simulink model "project"  (R2022b)
settings: Solver=FixedStepAuto  StartTime=0.0  StopTime=inf  RelTol=1e-3  EnableMultiTasking=on
libraries: arduinolib x10
settings Model: ExtModeTrigDuration=2  Creator=ESE  LastModifiedBy=ESE
settings OptimizationCC: EnhancedBackFolding=on  PassReuseOutputArgsAs=Individual arguments  ZeroExternalMemoryAtStartup=off  ZeroInternalMemoryAtStartup=off  MaxStackSize=64  OptimizeBlockOrder=speed  DifferentSizesBufferReuse=on  OptimizationCustomize=off  EfficientTunableParamExpr=on
settings DebuggingCC: ParameterTunabilityLossMsg=error
settings HardwareCC: ProdBitPerInt=16  ProdBitPerPointer=16  ProdBitPerSizeT=16  ProdBitPerPtrDiffT=16  ProdLargestAtomicFloat=None  ProdWordSize=8  ProdHWDeviceType=Atmel->AVR
settings SFSimCC: MATLABDynamicMemAlloc=off
settings RTWCC: Description=Embedded Coder  SystemTargetFile=ert.tlc  HardwareBoard=Arduino Mega 2560  TLCOptions=-aInlineSetEventsForThisBaseRateFcn=TLC_FALSE -aSuppressMultiTaskScheduler=TLC_FALSE -aRateBasedStepFcn=1  TemplateMakefile=ert_default_tmf  Toolchain=Arduino AVR  BuildConfiguration=Faster Runs
settings CodeAppCC: ForceParamTrailComments=on  IgnoreCustomStorageClasses=off  OperatorAnnotations=on  SimulinkDataObjDesc=on  SFDataObjDesc=on  InsertBlockDesc=on
settings ERTTargetCC: SupportContinuousTime=on  SupportVariableSizeSignals=on  ExtModeTransport=3  ExtModeStaticAlloc=on  ExtModeAutomaticAllocSize=off  ExtModeStaticAllocSize=2048  ExtModeMexFile=ext_xcp  ExtModeIntrfLevel=Level2 - Open

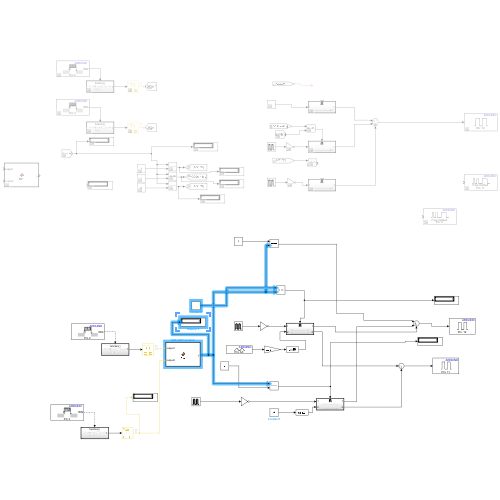
[thumbnail: Simulink's stored preview of the top-level diagram]
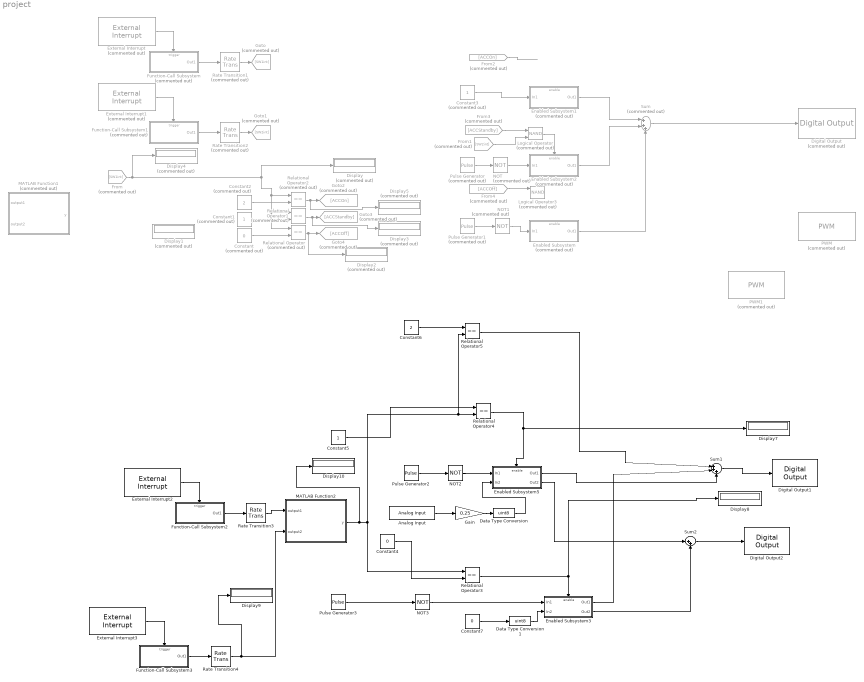
== system project ==
  Analog Input : arduinolib/Analog Input  pinNumber=0  ReadResultsOnly=off  ConversionTriggerSource=Software  ExternalTriggerType=uint32( 0 )  OutputDataType=uint16  EnableConversionCompleteNotify=off  EnableOuputStatus=off  SampleTime=-1  blockPlatform=arduino
  Constant : Constant  Commented=on  Value=0
  Constant1 : Constant  Commented=on
  Constant2 : Constant  Commented=on  Value=2
  Constant3 : Constant  Commented=on
  Constant4 : Constant  Value=0
  Constant5 : Constant
  Constant6 : Constant  Value=2
  Constant7 : Constant  Value=0
  Data Type Conversion : DataTypeConversion  OutDataTypeStr=uint8  SaturateOnIntegerOverflow=off  RndMeth=Floor
  Data Type Conversion1 : DataTypeConversion  OutDataTypeStr=uint8  SaturateOnIntegerOverflow=off  RndMeth=Floor
  Digital Output : arduinolib/Digital Output  Commented=on  pinNumber=12  Direction=output  blockPlatform=arduino
  Digital Output1 : arduinolib/Digital Output  pinNumber=12  Direction=output  blockPlatform=arduino
  Digital Output2 : arduinolib/Digital Output  pinNumber=11  Direction=output  blockPlatform=arduino
  Display{,1..5} (6 alike) : Display  Commented=on
  Display{7..10} (4 alike) : Display
  Enabled Subsystem : Subsystem  Commented=on  TreatAsAtomicUnit=on
  Enabled Subsystem1 : Subsystem  Commented=on  TreatAsAtomicUnit=on
  Enabled Subsystem2 : Subsystem  Commented=on  TreatAsAtomicUnit=on
  Enabled Subsystem3 : Subsystem  TreatAsAtomicUnit=on
  Enabled Subsystem5 : Subsystem  TreatAsAtomicUnit=on
  External Interrupt : arduinolib/External Interrupt  Commented=on  Pin=2  PullUp=off  Mode=FALLING  InterruptSimulationInput=off
  External Interrupt1 : arduinolib/External Interrupt  Commented=on  Pin=3  PullUp=off  Mode=FALLING  InterruptSimulationInput=off
  External Interrupt2 : arduinolib/External Interrupt  Pin=2  PullUp=off  Mode=FALLING  InterruptSimulationInput=off
  External Interrupt3 : arduinolib/External Interrupt  Pin=3  PullUp=off  Mode=FALLING  InterruptSimulationInput=off
  From : From  Commented=on  GotoTag=SW1int
  From1 : From  Commented=on  GotoTag=SW2int
  From2 : From  Commented=on  GotoTag=ACCOn
  From3 : From  Commented=on  GotoTag=ACCStandby
  From4 : From  Commented=on  GotoTag=ACCOff
  Function-Call Subsystem : Subsystem  Commented=on  TreatAsAtomicUnit=on
  Function-Call Subsystem1 : Subsystem  Commented=on  TreatAsAtomicUnit=on
  Function-Call Subsystem2 : Subsystem  TreatAsAtomicUnit=on
  Function-Call Subsystem3 : Subsystem  TreatAsAtomicUnit=on
  Gain : Gain  Gain=0.25
  Goto : Goto  Commented=on  GotoTag=SW1int
  Goto1 : Goto  Commented=on  GotoTag=SW2int
  Goto2 : Goto  Commented=on  GotoTag=ACCOn
  Goto3 : Goto  Commented=on  GotoTag=ACCStandby
  Goto4 : Goto  Commented=on  GotoTag=ACCOff
  Logical Operator : Logic  Commented=on  Operator=NAND  AllPortsSameDT=off  OutDataTypeStr=boolean
  Logical Operator3 : Logic  Commented=on  Operator=NAND  AllPortsSameDT=off  OutDataTypeStr=boolean
  MATLAB Function1 : MATLAB Function  Commented=on  TreatAsAtomicUnit=on
  MATLAB Function2 : MATLAB Function  TreatAsAtomicUnit=on
  NOT : Logic  Commented=on  Operator=NOT  IconShape=distinctive  AllPortsSameDT=off  OutDataTypeStr=boolean
  NOT1 : Logic  Commented=on  Operator=NOT  IconShape=distinctive  AllPortsSameDT=off  OutDataTypeStr=boolean
  NOT2 : Logic  Operator=NOT  IconShape=distinctive  AllPortsSameDT=off  OutDataTypeStr=boolean
  NOT3 : Logic  Operator=NOT  IconShape=distinctive  AllPortsSameDT=off  OutDataTypeStr=boolean
  PWM : arduinolib/PWM  Commented=on  pinNumber=11  frequencyType=Default  desiredFrequency=490.2  achievableFrequency=490.2
  PWM1 : arduinolib/PWM  Commented=on  pinNumber=8  frequencyType=Default  desiredFrequency=490.2  achievableFrequency=490.2
  Pulse Generator : DiscretePulseGenerator  Commented=on  PulseType=Time based  Period=0.4  PulseWidth=50
  Pulse Generator1 : DiscretePulseGenerator  Commented=on  PulseType=Time based  Period=0.4  PulseWidth=50
  Pulse Generator2 : DiscretePulseGenerator  PulseType=Time based  Period=0.4  PulseWidth=50
  Pulse Generator3 : DiscretePulseGenerator  PulseType=Time based  Period=0.4  PulseWidth=50
  Rate Transition1 : RateTransition  Commented=on  Deterministic=off
  Rate Transition2 : RateTransition  Commented=on  Deterministic=off
  Rate Transition3 : RateTransition  Deterministic=off
  Rate Transition4 : RateTransition  Deterministic=off
  Relational Operator : RelationalOperator  Commented=on  Operator===  OutDataTypeStr=boolean  RndMeth=Simplest  InputSameDT=off
  Relational Operator1 : RelationalOperator  Commented=on  Operator===  OutDataTypeStr=boolean  RndMeth=Simplest  InputSameDT=off
  Relational Operator2 : RelationalOperator  Commented=on  Operator===  OutDataTypeStr=boolean  RndMeth=Simplest  InputSameDT=off
  Relational Operator3 : RelationalOperator  Operator===  OutDataTypeStr=boolean  RndMeth=Simplest  InputSameDT=off
  Relational Operator4 : RelationalOperator  Operator===  OutDataTypeStr=boolean  RndMeth=Simplest  InputSameDT=off
  Relational Operator5 : RelationalOperator  Operator===  OutDataTypeStr=boolean  RndMeth=Simplest  InputSameDT=off
  Sum : Sum  Commented=on  Inputs=|+++
  Sum1 : Sum  Inputs=|+++
  Sum2 : Sum  Inputs=|++
  wires:
  Rate Transition1/1 -> Goto/1
  Enabled Subsystem/1(Out1) -> Sum/3
  Function-Call Subsystem/1(Out1) -> Rate Transition1/1
  External Interrupt/1 -> Function-Call Subsystem/Trigger
  Constant3/1 -> Enabled Subsystem1/1(In1)
  Sum/1 -> Digital Output/1
  Pulse Generator1/1 -> NOT1/1
  Constant/1 -> Relational Operator/2
  Constant2/1 -> Relational Operator2/2
  Function-Call Subsystem1/1(Out1) -> Rate Transition2/1
  External Interrupt1/1 -> Function-Call Subsystem1/Trigger
  Relational Operator1/1 -> Display3/1, Goto3/1
  Relational Operator2/1 -> Display5/1, Goto2/1
  NOT/1 -> Enabled Subsystem2/1(In1)
  From/1 -> Relational Operator2/1, Relational Operator/1, Relational Operator1/1, Display/1, Display4/1
  NOT1/1 -> Enabled Subsystem/1(In1)
  Pulse Generator/1 -> NOT/1
  Rate Transition2/1 -> Goto1/1
  Relational Operator/1 -> Display2/1, Goto4/1
  Constant1/1 -> Relational Operator1/2
  From3/1 -> Logical Operator/1
  From1/1 -> Logical Operator/2
  Logical Operator/1 -> Enabled Subsystem2/Enable
  From2/1 -> ?
  Enabled Subsystem1/1(Out1) -> Sum/1
  Enabled Subsystem2/1(Out1) -> Sum/2
  From4/1 -> Logical Operator3/1
  Relational Operator4/1 -> Enabled Subsystem5/Enable, Display7/1
  Enabled Subsystem5/1(Out1) -> Sum1/3
  Constant4/1 -> Relational Operator3/2
  Constant5/1 -> Relational Operator4/1
  Pulse Generator2/1 -> NOT2/1
  Sum1/1 -> Digital Output1/1
  NOT2/1 -> Enabled Subsystem5/1(In1)
  Pulse Generator3/1 -> NOT3/1
  Enabled Subsystem3/1(Out1) -> Sum1/2
  Function-Call Subsystem2/1(Out1) -> Rate Transition3/1
  External Interrupt2/1 -> Function-Call Subsystem2/Trigger
  Relational Operator3/1 -> Display8/1, Enabled Subsystem3/Enable
  Constant6/1 -> Relational Operator5/1
  NOT3/1 -> Enabled Subsystem3/1(In1)
  Relational Operator5/1 -> Sum1/1
  Function-Call Subsystem3/1(Out1) -> Rate Transition4/1
  External Interrupt3/1 -> Function-Call Subsystem3/Trigger
  Rate Transition4/1 -> Display9/1, MATLAB Function2/2(output2)
  Rate Transition3/1 -> MATLAB Function2/1(output1)
  MATLAB Function2/1(y) -> Display10/1, Relational Operator5/2, Relational Operator4/2, Relational Operator3/1
  Gain/1 -> Data Type Conversion/1
  Analog Input/1 -> Gain/1
  Data Type Conversion/1 -> Enabled Subsystem5/2(In2)
  Enabled Subsystem5/2(Out2) -> Sum2/1
  Sum2/1 -> Digital Output2/1
  Enabled Subsystem3/2(Out2) -> Sum2/2
  Constant7/1 -> Data Type Conversion1/1
  Data Type Conversion1/1 -> Enabled Subsystem3/2(In2)

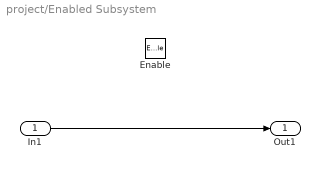
== system project/Enabled Subsystem ==
  In1 : Inport
  Enable : EnablePort  StatesWhenEnabling=reset
  Out1 : Outport
  wires:
  In1/1 -> Out1/1

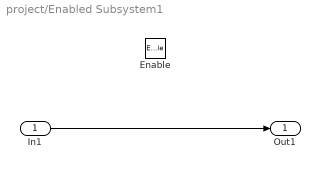
== system project/Enabled Subsystem1 ==
  In1 : Inport
  Enable : EnablePort
  Out1 : Outport
  wires:
  In1/1 -> Out1/1

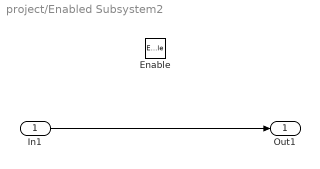
== system project/Enabled Subsystem2 ==
  In1 : Inport
  Enable : EnablePort
  Out1 : Outport
  wires:
  In1/1 -> Out1/1

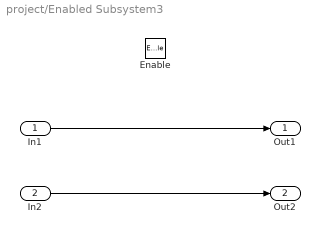
== system project/Enabled Subsystem3 ==
  In1 : Inport
  In2 : Inport  Port=2
  Enable : EnablePort  StatesWhenEnabling=reset
  Out1 : Outport
  Out2 : Outport  Port=2
  wires:
  In1/1 -> Out1/1
  In2/1 -> Out2/1

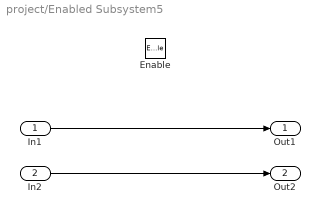
== system project/Enabled Subsystem5 ==
  In1 : Inport
  In2 : Inport  Port=2
  Enable : EnablePort
  Out1 : Outport
  Out2 : Outport  Port=2
  wires:
  In1/1 -> Out1/1
  In2/1 -> Out2/1

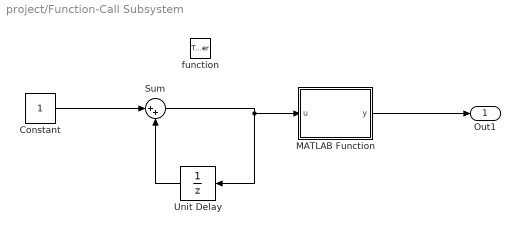
== system project/Function-Call Subsystem ==
  function : TriggerPort  TriggerType=function-call  VariantControl=(inherit)
  Constant : Constant
  MATLAB Function : MATLAB Function  TreatAsAtomicUnit=on
  Sum : Sum  Inputs=|++
  Unit Delay : UnitDelay  SampleTime=-1  HasFrameUpgradeWarning=on
  Out1 : Outport
  wires:
  Constant/1 -> Sum/1
  Unit Delay/1 -> Sum/2
  Sum/1 -> Unit Delay/1, MATLAB Function/1(u)
  MATLAB Function/1(y) -> Out1/1

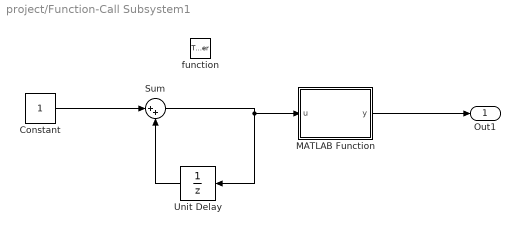
== system project/Function-Call Subsystem1 ==
  function : TriggerPort  TriggerType=function-call  VariantControl=(inherit)
  Constant : Constant
  MATLAB Function : MATLAB Function  TreatAsAtomicUnit=on
  Sum : Sum  Inputs=|++
  Unit Delay : UnitDelay  SampleTime=-1  HasFrameUpgradeWarning=on
  Out1 : Outport
  wires:
  Constant/1 -> Sum/1
  Unit Delay/1 -> Sum/2
  Sum/1 -> Unit Delay/1, MATLAB Function/1(u)
  MATLAB Function/1(y) -> Out1/1

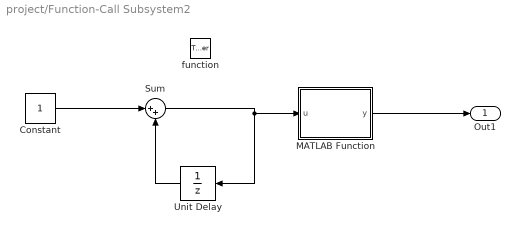
== system project/Function-Call Subsystem2 ==
  function : TriggerPort  TriggerType=function-call  VariantControl=(inherit)
  Constant : Constant
  MATLAB Function : MATLAB Function  TreatAsAtomicUnit=on
  Sum : Sum  Inputs=|++
  Unit Delay : UnitDelay  SampleTime=-1  HasFrameUpgradeWarning=on
  Out1 : Outport
  wires:
  Constant/1 -> Sum/1
  Unit Delay/1 -> Sum/2
  Sum/1 -> Unit Delay/1, MATLAB Function/1(u)
  MATLAB Function/1(y) -> Out1/1

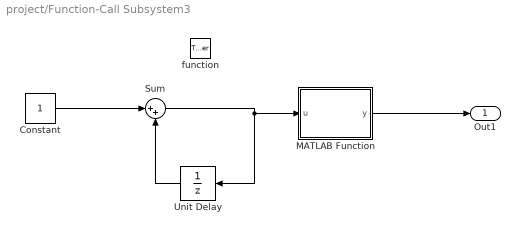
== system project/Function-Call Subsystem3 ==
  function : TriggerPort  TriggerType=function-call  VariantControl=(inherit)
  Constant : Constant
  MATLAB Function : MATLAB Function  TreatAsAtomicUnit=on
  Sum : Sum  Inputs=|++
  Unit Delay : UnitDelay  SampleTime=-1  HasFrameUpgradeWarning=on
  Out1 : Outport
  wires:
  Constant/1 -> Sum/1
  Unit Delay/1 -> Sum/2
  Sum/1 -> Unit Delay/1, MATLAB Function/1(u)
  MATLAB Function/1(y) -> Out1/1

== matlab function project/Function-Call Subsystem/MATLAB Function ==
  data: u input; y output
function y = fcn(u)
 rem = mod(u,3);

 if rem == 0
     y=0; %off
 elseif rem==1
     y=1; %ACC standard
 else 
     y=2; %ACC on
 end

 if u > 100
     u = 1;
 end

== matlab function project/Function-Call Subsystem2/MATLAB Function ==
  data: u input; y output
function y = fcn(u)
 rem = mod(u,3);

 if rem == 0
     y=0; %off
 elseif rem==1
     y=1; %ACC standard
 else 
     y=2; %ACC on
 end

 if u > 100
     u = 1;
 end

== matlab function project/MATLAB Function1 ==
  data: output1 input; y output; output2 input
function y = fcn(output1,output2)
if output2==0
    y=output1;
else
    y=0;
end

== matlab function project/Function-Call Subsystem3/MATLAB Function ==
  data: u input; y output
function y = fcn(u)
 rem = mod(u,2);

 if rem == 0
     y=0; %off
 else 
     y=1; %ACC on
 end

 if u > 100
     u = 1;
 end

== matlab function project/MATLAB Function2 ==
  data: output1 input; y output; output2 input
function y = fcn(output1,output2)
if output2==0
    y=output1;
else
    y=0;
end

== matlab function project/Function-Call Subsystem1/MATLAB Function ==
  data: u input; y output
function y = fcn(u)
 rem = mod(u,2);

 if rem == 0
     y=0; %off
 else 
     y=1; %ACC on
 end

 if u > 100
     u = 1;
 end
